simulink model "fengchangshuchuceyan"  (Simulink 7.4)
settings: Solver=ode45  StartTime=0.0  StopTime=100  RelTol=1e-3
libraries: powerlib x5
settings Model: Creator=admini  LastModifiedBy=admini

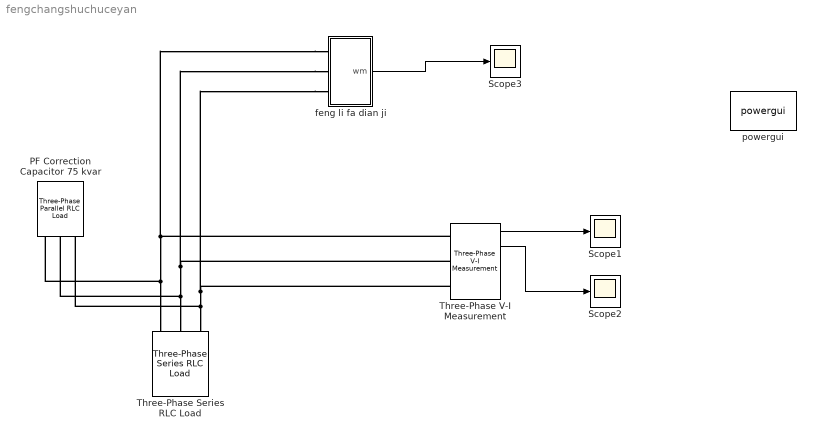
== system fengchangshuchuceyan ==
  PF Correction Capacitor 75 kvar : powerlib/Elements/Three-Phase Parallel RLC Load  DialogController=POWERSYS.PowerSysDialog  PhysicalDomain=powersysdomain  SubClassName=unknown  LeftPortType=p1  RightPortType=p1  LConnTagsString=A|B|C  Configuration=Delta  NominalVoltage=690  NominalFrequency=50  ActivePower=0  InductivePower=0  CapacitivePower=75e3  Measurements=None
  Scope1 : Scope
      settings: TimeRange=10  YMin=-90000  YMax=90000
  Scope2 : Scope
      settings: TimeRange=0.1  YMin=-6e-012  YMax=6e-012
  Scope3 : Scope
      settings: TimeRange=0.2999999999999972  YMin=2.175  YMax=2.22  SaveName=ScopeData2
  Three-Phase Series RLC Load : powerlib/Elements/Three-Phase Series RLC Load  DialogController=POWERSYS.PowerSysDialog  PhysicalDomain=powersysdomain  SubClassName=unknown  LeftPortType=p1  RightPortType=p1  LConnTagsString=A|B|C  Configuration=Y (grounded)  NominalVoltage=690  NominalFrequency=50  ActivePower=10e3  InductivePower=100  CapacitivePower=100  Measurements=None
  Three-Phase V-I Measurement : powerlib/Measurements/Three-Phase V-I Measurement  DialogController=POWERSYS.PowerSysDialog  SystemSampleTime=-1  VoltageMeasurement=phase-to-ground  SetLabelV=off  LabelV=Vabc  Vpu=off  CurrentMeasurement=yes  SetLabelI=off  LabelI=Iabc  Ipu=off  Pbase=100e6  Vbase=500e3  OutputType=Complex  PhasorSimulation=off  PSBequivalent=0
  feng li fa dian ji : Subsystem
  powergui : powerlib/powergui  Priority=1  SystemSampleTime=-1  SimulationMode=Continuous  SampleTime=50e-6  frequency=60  SPID=off  DisableSnubberDevices=off  DisableRonSwitches=off  DisableVfSwitches=off  SwTol=0  Interpol=off  frequencyindice=50  echomessages=off  HookPort=off  DisplayEquations=off  FunctionMessages=off  EnableUseOfTLC=off  x0status=blocks  RestoreLinks=warning  Frange=[0:2:500]  Ylog=off  Xlog=on  ShowGrid=off  save=off  variable=ZData  ZoomFFT=on  StartTime=0.0  cycles=1  DisplayStyle=1  fundamental=60  FreqAxis=off  MaxFrequency=1000  frequencyindicesteady=1  RmsSteady=1  display=off  Ts=0  methode=off
  wires:
  Three-Phase V-I Measurement/1 -> Scope1/1
  Three-Phase V-I Measurement/2 -> Scope2/1
  feng li fa dian ji/1(wm) -> Scope3/1
  connections:
  feng li fa dian ji/LConn1 -- Three-Phase V-I Measurement/LConn1 -- Three-Phase Series RLC Load/LConn1 -- PF Correction Capacitor 75 kvar/LConn1
  feng li fa dian ji/LConn2 -- Three-Phase V-I Measurement/LConn2 -- Three-Phase Series RLC Load/LConn2 -- PF Correction Capacitor 75 kvar/LConn2
  feng li fa dian ji/LConn3 -- Three-Phase V-I Measurement/LConn3 -- Three-Phase Series RLC Load/LConn3 -- PF Correction Capacitor 75 kvar/LConn3

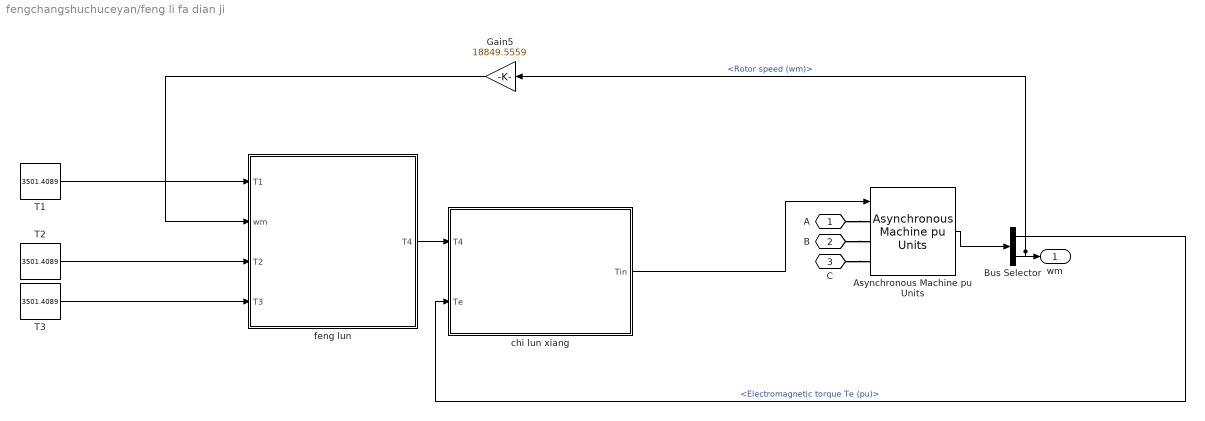
== system fengchangshuchuceyan/feng li fa dian ji ==
  Asynchronous Machine pu Units : powerlib/Machines/Asynchronous Machine pu Units  DialogController=POWERSYS.PowerSysDialog  SystemSampleTime=-1  PresetModel=No  MechanicalLoad=Torque Tm  ShowDetailedParameters=on  RotorType=Squirrel-cage  ReferenceFrame=Rotor  NominalParameters=[0.5e6 690 50]  Stator=[0.01965 0.0397]  Rotor=[0.01909 0.0397]  Lm=1.354  Mechanical=[0.1419 0.01 2]  PolePairs=2  InitialConditions="[ 1,0   1,1,1  0,0,0 ]"  Units=pu  LoadFlowParameters=0  SimulateSaturation=off  Saturation="[0.212,0.4201,0.8125,1.0979,1.4799,2.2457,3.2586,4.5763,6.4763 ;   0.5,0.7,0.9,1,1.1,1.2 ,1.3,1.4,1.5]"  TsPowergui=0  TsBlock=-1  IterativeModel=Forward Euler
      link override Electrical model/Continuous/Stator/phiqs: InitialCondition=0.00001
      link override Mechanical model/Continuous Tm input/Rotor angle thetam: InitialCondition=0.0001
      link override Mechanical model/Continuous Tm input/Rotor speed (wm): InitialCondition=0.0001
  Bus Selector : BusSelector  OutputSignals=Mechanical.Electromagnetic torque Te (pu),Mechanical.Rotor speed (wm)
  Gain5 : Gain  Gain=18849.5559  ParameterDataType=fixdt(1, 16)  ParameterScaling=2^0  OutDataType=fixdt(1, 16)  OutScaling=2^0
  T1 : Constant  Value=3501.4089  OutDataType=fixdt(1, 16)  OutScaling=2^0
  T2 : Constant  Value=3501.4089  OutDataType=fixdt(1, 16)  OutScaling=2^0
  T3 : Constant  Value=3501.4089  OutDataType=fixdt(1, 16)  OutScaling=2^0
  chi lun xiang : Subsystem
  feng lun : Subsystem
  A : PMIOPort  Port=1  Side=Left
  B : PMIOPort  Port=2  Side=Left
  C : PMIOPort  Port=3  Side=Left
  wm : Outport
  wires:
  Asynchronous Machine pu Units/1 -> Bus Selector/1
  Bus Selector/2 -> Gain5/1, wm/1  "<Rotor speed (wm)>"
  chi lun xiang/1(Tin) -> Asynchronous Machine pu Units/1
  feng lun/1(T4) -> chi lun xiang/1(T4)
  Bus Selector/1 -> chi lun xiang/2(Te)  "<Electromagnetic torque Te (pu)>"
  T2/1 -> feng lun/3(T2)
  T3/1 -> feng lun/4(T3)
  T1/1 -> feng lun/1(T1)
  Gain5/1 -> feng lun/2(wm)
  connections:
  A/RConn1 -- Asynchronous Machine pu Units/LConn1
  B/RConn1 -- Asynchronous Machine pu Units/LConn2
  C/RConn1 -- Asynchronous Machine pu Units/LConn3

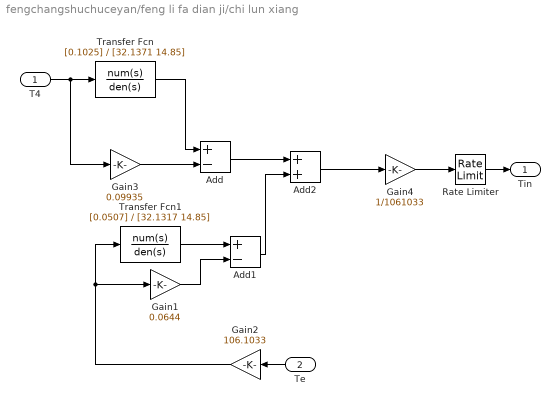
== system fengchangshuchuceyan/feng li fa dian ji/chi lun xiang ==
  T4 : Inport
  Te : Inport  Port=2
  Add : Sum  Inputs=+-  OutDataType=fixdt(1, 16)  OutScaling=2^-10
  Add1 : Sum  Inputs=+-  OutDataType=fixdt(1, 16)  OutScaling=2^-10
  Add2 : Sum  OutDataType=fixdt(1, 16)  OutScaling=2^-10
  Gain1 : Gain  Gain=0.0644  ParameterDataType=fixdt(1, 16)  ParameterScaling=2^0  OutDataType=fixdt(1, 16)  OutScaling=2^0
  Gain2 : Gain  Gain=106.1033  ParameterDataType=fixdt(1, 16)  ParameterScaling=2^0  OutDataType=fixdt(1, 16)  OutScaling=2^0
  Gain3 : Gain  Gain=0.09935  ParameterDataType=fixdt(1, 16)  ParameterScaling=2^0  OutDataType=fixdt(1, 16)  OutScaling=2^0
  Gain4 : Gain  Gain=1/1061033  ParameterDataType=fixdt(1, 16)  ParameterScaling=2^0  OutDataType=fixdt(1, 16)  OutScaling=2^0
  Rate Limiter : RateLimiter  RisingSlewLimit=10000  FallingSlewLimit=-10000  SampleTimeMode=inherited
  Transfer Fcn : TransferFcn  Numerator=[0.1025]  Denominator=[32.1371 14.85]  AbsoluteTolerance=0.001
  Transfer Fcn1 : TransferFcn  Numerator=[0.0507]  Denominator=[32.1317 14.85]
  Tin : Outport
  wires:
  Transfer Fcn/1 -> Add/1
  Transfer Fcn1/1 -> Add1/1
  Add/1 -> Add2/1
  Add1/1 -> Add2/2
  Gain3/1 -> Add/2
  Gain1/1 -> Add1/2
  Gain2/1 -> Transfer Fcn1/1, Gain1/1
  Add2/1 -> Gain4/1
  Gain4/1 -> Rate Limiter/1
  T4/1 -> Gain3/1, Transfer Fcn/1
  Rate Limiter/1 -> Tin/1
  Te/1 -> Gain2/1

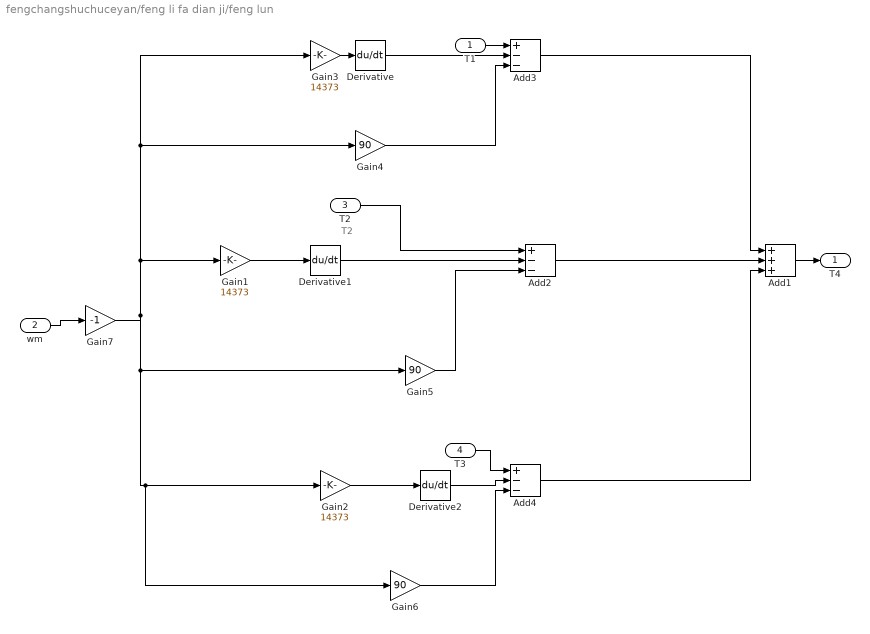
== system fengchangshuchuceyan/feng li fa dian ji/feng lun ==
  note: T2
  T1 : Inport
  wm : Inport  Port=2  OutDataType=fixdt(1, 16)  OutScaling=2^0
  T2 : Inport  Port=3
  T3 : Inport  Port=4
  Add1 : Sum  Inputs=+++  OutDataType=fixdt(1, 16)  OutScaling=2^-10
  Add2 : Sum  Inputs=+--  OutDataType=fixdt(1, 16)  OutScaling=2^-10
  Add3 : Sum  Inputs=+--  OutDataType=fixdt(1, 16)  OutScaling=2^-10
  Add4 : Sum  Inputs=+--  OutDataType=fixdt(1, 16)  OutScaling=2^-10
  Derivative : Derivative
  Derivative1 : Derivative
  Derivative2 : Derivative
  Gain1 : Gain  Gain=14373  ParameterDataType=fixdt(1, 16)  ParameterScaling=2^0  OutDataType=fixdt(1, 16)  OutScaling=2^0
  Gain2 : Gain  Gain=14373  ParameterDataType=fixdt(1, 16)  ParameterScaling=2^0  OutDataType=fixdt(1, 16)  OutScaling=2^0
  Gain3 : Gain  Gain=14373  ParameterDataType=fixdt(1, 16)  ParameterScaling=2^0  OutDataType=fixdt(1, 16)  OutScaling=2^0
  Gain4 : Gain  Gain=90  ParameterDataType=fixdt(1, 16)  ParameterScaling=2^0  OutDataType=fixdt(1, 16)  OutScaling=2^0
  Gain5 : Gain  Gain=90  ParameterDataType=fixdt(1, 16)  ParameterScaling=2^0  OutDataType=fixdt(1, 16)  OutScaling=2^0
  Gain6 : Gain  Gain=90  ParameterDataType=fixdt(1, 16)  ParameterScaling=2^0  OutDataType=fixdt(1, 16)  OutScaling=2^0
  Gain7 : Gain  Gain=-1  ParameterDataType=fixdt(1, 16)  ParameterScaling=2^0  OutDataType=fixdt(1, 16)  OutScaling=2^0
  T4 : Outport
  wires:
  Add3/1 -> Add1/1
  Add4/1 -> Add1/3
  Gain3/1 -> Derivative/1
  Derivative/1 -> Add3/2
  Gain1/1 -> Derivative1/1
  Gain2/1 -> Derivative2/1
  Derivative2/1 -> Add4/2
  Add2/1 -> Add1/2
  Gain4/1 -> Add3/3
  Gain6/1 -> Add4/3
  Add1/1 -> T4/1
  Gain7/1 -> Gain1/1, Gain3/1, Gain4/1, Gain2/1, Gain6/1, Gain5/1
  wm/1 -> Gain7/1
  T1/1 -> Add3/1
  T3/1 -> Add4/1
  T2/1 -> Add2/1
  Derivative1/1 -> Add2/2
  Gain5/1 -> Add2/3
